simulink model "LD3D"  (Simulink 7.2)
settings: Solver=ode45  StartTime=0.0  StopTime=43  RelTol=1e-3
undefined symbols (not defined in the file or in its folder): Poz, Vel
settings Model: Creator=derkachow  LastModifiedBy=derkachow  SimulationMode=accelerator
settings DataIOCC: SaveTime=off
settings OptimizationCC: InitFltsAndDblsToZero=on
settings DebuggingCC: SaveWithParameterizedLinksMsg=none  SignalResolutionControl=TryResolveAllWithWarning  MultiTaskDSMMsg=warning  MultiTaskCondExecSysMsg=none
settings RTWCC: IncludeERTFirstTime=on
settings GRTTargetCC: TargetFcnLib=ansi_tfl_tmw.mat

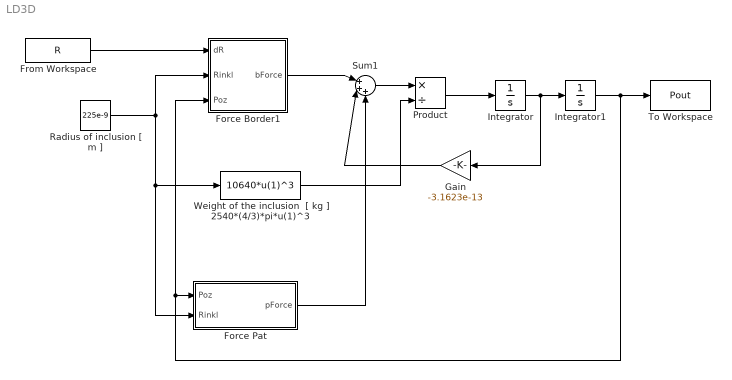
== system LD3D ==
  Force Border1 : Stateflow chart
  Force Pat : Stateflow chart
  From Workspace : FromWorkspace  VariableName=R  SampleTime=0
  Gain : Gain  Orientation=left  Gain=-3.1623e-13  ParameterDataType=sfix(16)  ParameterScaling=2^0  OutDataType=sfix(16)  OutScaling=2^0
  Integrator : Integrator  InitialCondition=Vel
  Integrator1 : Integrator  InitialCondition=Poz
  Product : Product  Inputs=*/  OutDataType=sfix(16)  OutScaling=2^0  RndMeth=Zero
  Radius of inclusion [ m ] : Constant  Value=225e-9  OutDataType=sfix(16)  OutScaling=2^0
  Sum1 : Sum  Inputs=|+++  OutDataType=sfix(16)  OutScaling=2^0
  To Workspace : ToWorkspace  VariableName=Pout  SampleTime=0.01  SaveFormat=Structure With Time
  Weight of the inclusion  [ kg ] 2540*(4/3)*pi*u(1)^3 : Fcn  Expr=10640*u(1)^3
  wires:
  From Workspace/1 -> Force Border1/1(dR)
  Radius of inclusion [ m ]/1 -> Force Border1/2(Rinkl), Weight of the inclusion  [ kg ] 2540*(4/3)*pi*u(1)^3/1, Force Pat/2(Rinkl)
  Force Border1/1(bForce) -> Sum1/1
  Force Pat/1(pForce) -> Sum1/3
  Gain/1 -> Sum1/2
  Weight of the inclusion  [ kg ] 2540*(4/3)*pi*u(1)^3/1 -> Product/2
  Sum1/1 -> Product/1
  Product/1 -> Integrator/1
  Integrator/1 -> Integrator1/1, Gain/1
  Integrator1/1 -> To Workspace/1, Force Border1/3(Poz), Force Pat/1(Poz)

== matlab function Force Pat ==
  data: Poz input double; pForce output double; Rinkl input double
function pForce = fcn( Poz, Rinkl )
% The function fcn( Poz, Rinkl ) calculates the interaction forces between inclusions.
% Forces are calculated based on Lennard-Jones potential.
Cinkl = size(Poz,1);
pForce = zeros(Cinkl,3);
distx = 0;
disty = 0;
distz =0;
F1 = 0;
F2 = 0;
epsi = -1e-25;
for ii = 1 : Cinkl
    for jj = 1: Cinkl
        
        distx =  Poz(ii,1) - Poz(jj,1);
        disty =  Poz(ii,2) - Poz(jj,2);
        distz =  Poz(ii,3) - Poz(jj,3);
               
        if ii ~= jj
            F1 = - 6 * ( ( (2*Rinkl)^12 ) / ( distx^2 + disty^2 + distz^2 )^7 )*2*distx;
            F2 =   6 * ( ( (2*Rinkl)^6  ) / ( distx^2 + disty^2 + distz^2 )^4 )*2*distx;
            pForce( ii, 1 ) = pForce( ii, 1 ) + epsi*( F1 + F2 );

            F1 = - 6 * ( ( (2*Rinkl)^12 ) / ( distx^2 + disty^2 + distz^2 )^7 )*2*disty;
            F2 =   6 * ( ( (2*Rinkl)^6  ) / ( distx^2 + disty^2 + distz^2 )^4 )*2*disty;
            pForce( ii, 2 ) = pForce( ii, 2 ) + epsi*( F1 + F2 );
       
            F1 = - 6 * ( ( (2*Rinkl)^12 ) / ( distx^2 + disty^2 + distz^2)^7 )*2*distz;
            F2 =   6 * ( ( (2*Rinkl)^6  ) / ( distx^2 + disty^2 + distz^2)^4 )*2*distz;
            pForce( ii, 3 ) = pForce( ii, 3 ) + epsi*( F1 + F2 );


        end
    end
end

== matlab function Force Border1 ==
  data: dR input double; bForce output double; Rinkl input double; Poz input double
function bForce = fcn( dR, Rinkl, Poz )
% The function calculates the interaction between 
% particles and the moving droplet's surface. 
% The function mimics the surface tension through elastic force.  
Cinkl = size( Poz,1 );
bForce = zeros( Cinkl, 3 );
k =1e-10;
X = 0;
Y = 0;
Z = 0;
RHO = 0;
THETA = 0;
PHI = 0;
for ii = 1: Cinkl
    [THETA,PHI,RHO] = cart2sph( Poz(ii,1), Poz(ii,2), Poz(ii,3) );
      distance =  dR - RHO;
    if abs( distance ) <= Rinkl
        f = k*distance;
        [X,Y,Z] = sph2cart(THETA,PHI,f);
        bForce( ii,1 ) = X;
        bForce( ii,2 ) = Y;
        bForce( ii,3 ) = Z;
    end
end
